simulink model "pct_03_org"  (Simulink 10.0)
settings: Solver=ode45  StartTime=0.0  StopTime=10.0  RelTol=1e-3
settings Model: Creator=moeller  LastModifiedBy=bhisma
settings DataIOCC: LimitDataPoints=on
settings OptimizationCC: BlockReduction=off  BooleanDataType=off
settings DebuggingCC: SaveWithParameterizedLinksMsg=none  SignalResolutionControl=TryResolveAllWithWarning
settings HardwareCC: TargetUnknown=on
settings GRTTargetCC: GeneratePreprocessorConditionals=Disable all  CombineOutputUpdateFcns=on  GRTInterface=off
settings ConfigComp: CovExternalEMLEnable=off  CovSFcnEnable=off

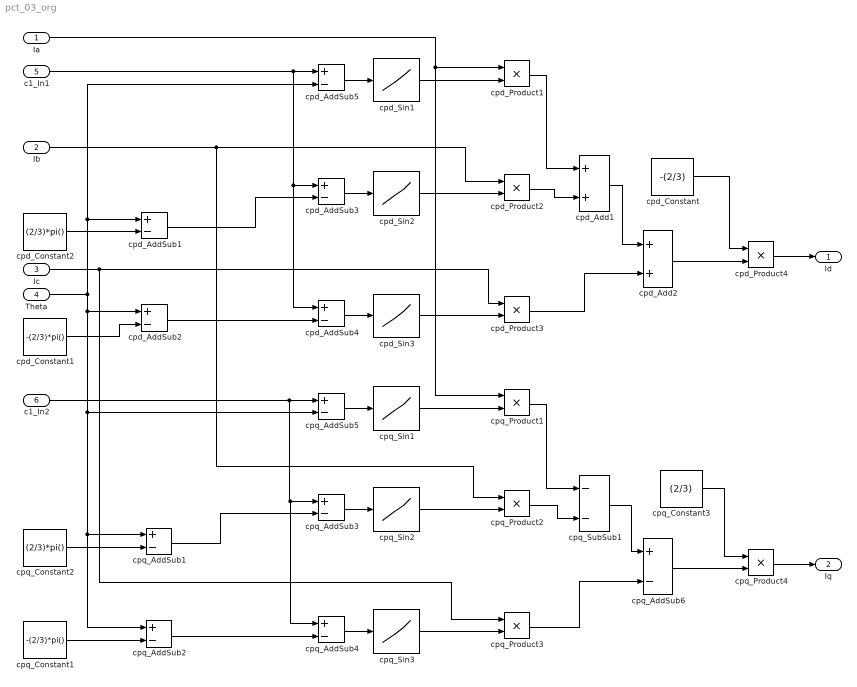
== system pct_03_org ==
  Ia : Inport  OutDataTypeStr=fixdt(1,16,4)
  Ib : Inport  Port=2  OutDataTypeStr=fixdt(1,16,4)
  Ic : Inport  Port=3  OutDataTypeStr=fixdt(1,16,4)
  Theta : Inport  Port=4  OutDataTypeStr=fixdt(1,16,4)
  c1_In1 : Inport  Port=5  OutDataTypeStr=fixdt(1,16,4)
  c1_In2 : Inport  Port=6  OutDataTypeStr=fixdt(1,16,4)
  cpd_Add1 : Sum  AccumDataTypeStr=fixdt(1,64,43)  OutDataTypeStr=fixdt(1,64,43)
  cpd_Add2 : Sum  AccumDataTypeStr=fixdt(1,64,43)  OutDataTypeStr=fixdt(1,64,43)
  cpd_AddSub{1..5} (5 alike) : Sum  Inputs=+-  AccumDataTypeStr=fixdt(1,16,4)  OutDataTypeStr=fixdt(1,16,4)
  cpd_Constant : Constant  Value=-(2/3)  OutDataTypeStr=Inherit: Inherit via back propagation
  cpd_Constant1 : Constant  Value=-(2/3)*pi()  OutDataTypeStr=Inherit: Inherit via back propagation
  cpd_Constant2 : Constant  Value=(2/3)*pi()  OutDataTypeStr=Inherit: Inherit via back propagation
  cpd_Product{1..4} (4 alike) : Product  OutDataTypeStr=fixdt(1,48,43)  RndMeth=Zero
  cpd_Sin1 : Lookup_n-D  NumberOfTableDimensions=1  BreakpointsForDimension1=[0:1024]  IndexSearchMethod=Evenly spaced points  BeginIndexSearchUsingPreviousIndexResult=on  Table=sin((0:1024))'  ExtrapMethod=Clip  DiagnosticForOutOfRangeInput=Warning  RemoveProtectionInput=on  UseLastTableValue=on  OutDataTypeStr=fixdt(1,16,15)  InputSameDT=on
  cpd_Sin2 : Lookup_n-D  NumberOfTableDimensions=1  BreakpointsForDimension1=[0:1024]  IndexSearchMethod=Evenly spaced points  BeginIndexSearchUsingPreviousIndexResult=on  Table=sin((0:1024))'  ExtrapMethod=Clip  DiagnosticForOutOfRangeInput=Warning  RemoveProtectionInput=on  UseLastTableValue=on  OutDataTypeStr=fixdt(1,16,15)  InputSameDT=on
  cpd_Sin3 : Lookup_n-D  NumberOfTableDimensions=1  BreakpointsForDimension1=[0:1024]  IndexSearchMethod=Evenly spaced points  BeginIndexSearchUsingPreviousIndexResult=on  Table=sin((0:1024))'  ExtrapMethod=Clip  DiagnosticForOutOfRangeInput=Warning  RemoveProtectionInput=on  UseLastTableValue=on  OutDataTypeStr=fixdt(1,16,15)  InputSameDT=on
  cpq_AddSub{1..5} (5 alike) : Sum  Inputs=+-  AccumDataTypeStr=fixdt(1,16,4)  OutDataTypeStr=fixdt(1,16,4)
  cpq_AddSub6 : Sum  Inputs=+-  AccumDataTypeStr=fixdt(1,64,43)  OutDataTypeStr=fixdt(1,64,43)
  cpq_Constant1 : Constant  Value=-(2/3)*pi()  OutDataTypeStr=Inherit: Inherit via back propagation
  cpq_Constant2 : Constant  Value=(2/3)*pi()  OutDataTypeStr=Inherit: Inherit via back propagation
  cpq_Constant3 : Constant  Value=(2/3)  OutDataTypeStr=Inherit: Inherit via back propagation
  cpq_Product{1..4} (4 alike) : Product  OutDataTypeStr=fixdt(1,48,43)  RndMeth=Zero
  cpq_Sin1 : Lookup_n-D  NumberOfTableDimensions=1  BreakpointsForDimension1=[0:1024]  IndexSearchMethod=Evenly spaced points  BeginIndexSearchUsingPreviousIndexResult=on  Table=sin((0:1024))'  ExtrapMethod=Clip  DiagnosticForOutOfRangeInput=Warning  RemoveProtectionInput=on  UseLastTableValue=on  OutDataTypeStr=fixdt(1,16,15)  InputSameDT=on
  cpq_Sin2 : Lookup_n-D  NumberOfTableDimensions=1  BreakpointsForDimension1=[0:1024]  IndexSearchMethod=Evenly spaced points  BeginIndexSearchUsingPreviousIndexResult=on  Table=sin((0:1024))'  ExtrapMethod=Clip  DiagnosticForOutOfRangeInput=Warning  RemoveProtectionInput=on  UseLastTableValue=on  OutDataTypeStr=fixdt(1,16,15)  InputSameDT=on
  cpq_Sin3 : Lookup_n-D  NumberOfTableDimensions=1  BreakpointsForDimension1=[0:1024]  IndexSearchMethod=Evenly spaced points  BeginIndexSearchUsingPreviousIndexResult=on  Table=sin((0:1024))'  ExtrapMethod=Clip  DiagnosticForOutOfRangeInput=Warning  RemoveProtectionInput=on  UseLastTableValue=on  OutDataTypeStr=fixdt(1,16,15)  InputSameDT=on
  cpq_SubSub1 : Sum  Inputs=--  AccumDataTypeStr=fixdt(1,64,43)  OutDataTypeStr=fixdt(1,64,43)
  Id : Outport
  Iq : Outport  Port=2
  wires:
  Ia/1 -> cpd_Product1/1, cpq_Product1/1
  Ib/1 -> cpd_Product2/1, cpq_Product2/1
  Ic/1 -> cpd_Product3/1, cpq_Product3/1
  cpd_Add1/1 -> cpd_Add2/1
  cpd_Add2/1 -> cpd_Product4/2
  cpd_Constant/1 -> cpd_Product4/1
  cpd_Constant1/1 -> cpd_AddSub2/2
  c1_In1/1 -> cpd_AddSub4/1, cpd_AddSub3/1, cpd_AddSub5/1
  cpd_Constant2/1 -> cpd_AddSub1/2
  cpd_Product4/1 -> Id/1
  cpd_Product1/1 -> cpd_Add1/1
  cpd_Product2/1 -> cpd_Add1/2
  cpd_Product3/1 -> cpd_Add2/2
  cpd_Sin1/1 -> cpd_Product1/2
  cpd_Sin2/1 -> cpd_Product2/2
  cpd_Sin3/1 -> cpd_Product3/2
  cpd_AddSub1/1 -> cpd_AddSub3/2
  cpd_AddSub2/1 -> cpd_AddSub4/2
  cpd_AddSub3/1 -> cpd_Sin2/1
  cpd_AddSub4/1 -> cpd_Sin3/1
  cpd_AddSub5/1 -> cpd_Sin1/1
  Theta/1 -> cpd_AddSub1/1, cpd_AddSub5/2, cpq_AddSub1/1, cpq_AddSub2/1, cpq_AddSub5/2, cpd_AddSub2/1
  cpq_SubSub1/1 -> cpq_AddSub6/1
  cpq_AddSub6/1 -> cpq_Product4/2
  cpq_Constant3/1 -> cpq_Product4/1
  cpq_Constant1/1 -> cpq_AddSub2/2
  c1_In2/1 -> cpq_AddSub4/1, cpq_AddSub3/1, cpq_AddSub5/1
  cpq_Constant2/1 -> cpq_AddSub1/2
  cpq_Product4/1 -> Iq/1
  cpq_Product1/1 -> cpq_SubSub1/1
  cpq_Product2/1 -> cpq_SubSub1/2
  cpq_Product3/1 -> cpq_AddSub6/2
  cpq_Sin1/1 -> cpq_Product1/2
  cpq_Sin2/1 -> cpq_Product2/2
  cpq_Sin3/1 -> cpq_Product3/2
  cpq_AddSub1/1 -> cpq_AddSub3/2
  cpq_AddSub2/1 -> cpq_AddSub4/2
  cpq_AddSub3/1 -> cpq_Sin2/1
  cpq_AddSub4/1 -> cpq_Sin3/1
  cpq_AddSub5/1 -> cpq_Sin1/1
